simulink model "work"  (R2020b)
settings: Solver=VariableStepAuto  StartTime=0.0  StopTime=100  RelTol=1e-3
settings Model: Creator=zhiyao  LastModifiedBy=zhiyao

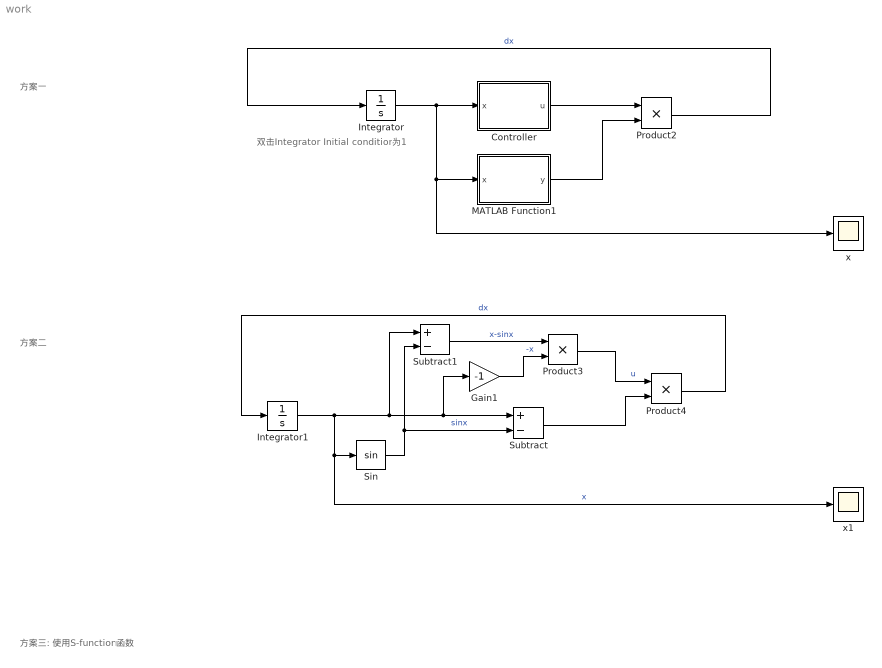
== system work ==
  note: 方案一
  note: 双击Integrator Initial condition为1
  note: 方案二
  note: 方案三: 使用S-function函数
  Controller : MATLAB Function  TreatAsAtomicUnit=on
  Gain1 : Gain  Gain=-1
  Integrator : Integrator  InitialCondition=1
  Integrator1 : Integrator  InitialCondition=1
  MATLAB Function1 : MATLAB Function  TreatAsAtomicUnit=on
  Product2 : Product
  Product3 : Product
  Product4 : Product
  Sin : Trigonometry
  Subtract : Sum  Inputs=+-
  Subtract1 : Sum  Inputs=+-
  x : Scope
  x1 : Scope
  wires:
  Integrator/1 -> x/1, MATLAB Function1/1(x), Controller/1(x)
  Controller/1(u) -> Product2/1
  MATLAB Function1/1(y) -> Product2/2
  Product2/1 -> Integrator/1  "dx"
  Integrator1/1 -> Subtract/1, Gain1/1, Subtract1/1, x1/1, Sin/1  "x"
  Sin/1 -> Subtract1/2, Subtract/2  "sinx"
  Subtract1/1 -> Product3/1  "x-sinx"
  Product3/1 -> Product4/1  "u"
  Gain1/1 -> Product3/2  "-x"
  Subtract/1 -> Product4/2
  Product4/1 -> Integrator1/1  "dx"

== matlab function work/MATLAB Function1 ==
  data: x input; y output
function y = fcn(x)

y = x-sin(x);

== matlab function work/Controller ==
  data: x input; u output
function u = fcn(x)

u = -x.*(x-sin(x));
